simulink model "sys_sim_whx"  (R2023b)
settings: Solver=ode45  StartTime=0.0  StopTime=30  FixedStep=0.001  MaxStep=0.001  MinStep=0.0001  RelTol=1e-3
model workspace (MAT data in the model file):
  Ld = 0.27
  Lu = 0.15
  Tj_MAX = 35
  Tw_MAX = 7
values from neighbouring files (symbols this model uses):
  eta_l = 0.4406    [sys_calc.m]    (also in sys_calc_whx.m = 0.3088)
  g = 9.80665    [sys_calc.m]    (also in sys_calc_whx.m)
  mb = 18.3393    [sys_calc.m]
  ml = 0.924    [sys_calc.m]
  N = NM + mp*diff(x + L*sin(theta),t,2)    [sys_calc_whx.m]
  Rl = 0.18    [sys_calc.m]
  Rw = 0.06    [sys_calc.m]
undefined symbols (not defined in the file or in its folder): X, Y, Z
libraries: sm_lib x76, nesl_utility x38, simulink x9, slpidlib x4
(part 1 of 4)
settings Model: SimulationMode=accelerator  Creator=XH  LastModifiedBy=XHServer
settings DataIOCC: ReturnWorkspaceOutputs=off
settings OptimizationCC: ReuseModelBlockBuffer=off
settings DebuggingCC: ReadBeforeWriteMsg=DisableAll  WriteAfterWriteMsg=DisableAll  WriteAfterReadMsg=DisableAll  MultiTaskDSMMsg=none
settings ModelReferenceCC: UpdateModelReferenceTargets=IfOutOfDate  EnableParallelModelReferenceBuilds=on
settings SFSimCC: SFSimEcho=off  SimTargetLang=C++
settings ExplorerConfigSet: InternalSimMechanicsExplorerSettings="<ExplorerConfiguration><canonicalview>planar_xy</canonicalview><AnimationSetting><BasePlaybackSpeed>1.0</BasePlaybackSpeed><PlaybackSpeedFactor>1.0</PlaybackSpeedFactor></AnimationSetting><TilePanel><TileInfo><Tiles Columns=\"1\" Count=\"1\" Rows=\"1\"><Column Weight=\"1\"/><Row Weight=\"1\"/><Tile Height=\"1\" Width=\"1\" X=\"0\" Y=\"0\"/></Tiles></TileInfo><SceneInfo><SceneViewer><BGColor><R>0.60000002384185791</R><G>0.60000002384185791</G><B>0.60000002384185791</B></BGColor><Camera><DoPerspective>off</DoPerspective><Position><X>8.61621392892213223</X><Y>7.77837481059580949</Y><Z>8.14104102643142014</Z></Position><Center><X>0.437671063196747923</X><Y>-0.400168055129575428</Y><Z>-0.0375018392939591994</Z></Center><Up><X>-0.408248290463863073</X><Y>0.816496580927726145</Y><Z>-0.408248290463863073</Z></Up><ViewLimDist>1</ViewLimDist><YLim>4.22529414972195827</YLim><XLim>7.13870261586088883</XLim></Camera></SceneViewer></SceneInfo></TilePanel><MechEditorPanel><Cameras/><GfxPanelCameraMap/><VideoCreator><PlaybackSpeedRatio>1.0</PlaybackSpeedRatio><FrameRate>30</FrameRate><VideoFormat>Motion JPEG AVI</VideoFormat><FrameSize>auto</FrameSize></VideoCreator></MechEditorPanel></ExplorerConfiguration>"

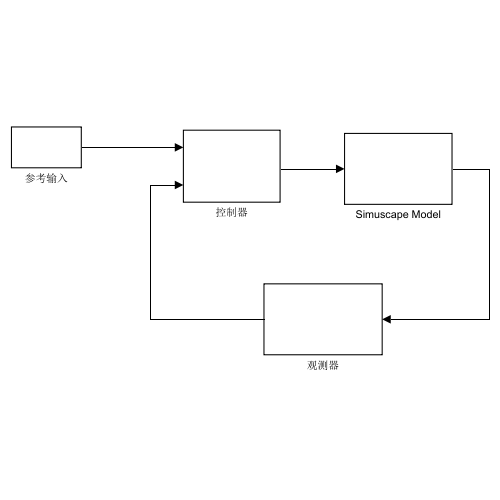
[thumbnail: Simulink's stored preview of the top-level diagram]
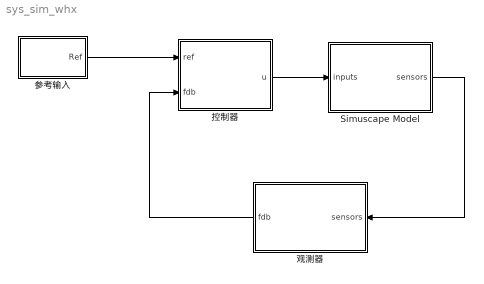
== system sys_sim_whx ==
  Simuscape Model : Subsystem
  参考输入 : Subsystem
  控制器 : Subsystem
  观测器 : Subsystem
  wires:
  Simuscape Model/1(sensors) -> 观测器/1(sensors)
  观测器/1(fdb) -> 控制器/2(fdb)
  参考输入/1(Ref) -> 控制器/1(ref)
  控制器/1(u) -> Simuscape Model/1(inputs)

== system sys_sim_whx/Simuscape Model ==
  inputs : Inport
  Bus Creator : BusCreator  Inputs=28
  Bus Selector1 : BusSelector  OutputSignals=T_lwl,T_lwr,T_Jl1,T_Jl2,T_Jr1,T_Jr2
  Physical System : Subsystem
  sensors : Outport
  wires:
  Bus Selector1/5 -> Physical System/5(T_Jr1)  "<T_Jr1>"
  Bus Selector1/6 -> Physical System/6(T_Jr2)  "<T_Jr2>"
  Bus Selector1/4 -> Physical System/4(T_Jl2)  "<T_Jl2>"
  Bus Selector1/3 -> Physical System/3(T_Jl1)  "<T_Jl1>"
  Bus Selector1/1 -> Physical System/1(T_lwl)  "<T_lwl>"
  Bus Selector1/2 -> Physical System/2(T_lwr)  "<T_lwr>"
  Bus Creator/1 -> sensors/1
  inputs/1 -> Bus Selector1/1
  Physical System/17(Φd) -> Bus Creator/17  "Φd"
  Physical System/16(Φ) -> Bus Creator/16  "Φ"
  Physical System/15(θ_wr) -> Bus Creator/15  "θ_wr"
  Physical System/14(θ_wrd) -> Bus Creator/14  "θ_wrd"
  Physical System/13(θ_wl) -> Bus Creator/13  "θ_wl"
  Physical System/12(θ_wld) -> Bus Creator/12  "θ_wld"
  Physical System/11(θ_Jr2) -> Bus Creator/11  "θ_Jr2"
  Physical System/10(θ_Jr1) -> Bus Creator/10  "θ_Jr1"
  Physical System/9(θ_Jl2) -> Bus Creator/9  "θ_Jl2"
  Physical System/8(θ_Jl1) -> Bus Creator/8  "θ_Jl1"
  Physical System/7(lr) -> Bus Creator/7  "lr"
  Physical System/6(θ_blr) -> Bus Creator/6  "θ_blr"
  Physical System/5(ll) -> Bus Creator/5  "ll"
  Physical System/4(θ_bll) -> Bus Creator/4  "θ_bll"
  Physical System/3(ψ) -> Bus Creator/3  "ψ"
  Physical System/2(θ_bd) -> Bus Creator/2  "θ_bd"
  Physical System/1(θ_b) -> Bus Creator/1  "θ_b"
  Physical System/18(s) -> Bus Creator/18  "s"
  Physical System/19(sd) -> Bus Creator/19  "sd"
  Physical System/20(az) -> Bus Creator/20  "az"
  Physical System/21(Tr1) -> Bus Creator/21  "Tr1"
  Physical System/22(Tr2) -> Bus Creator/22  "Tr2"
  Physical System/23(Tl1) -> Bus Creator/23  "Tl1"
  Physical System/24(Tl2) -> Bus Creator/24  "Tl2"
  Physical System/25(θd_Jr1) -> Bus Creator/25  "θd_Jr1"
  Physical System/26(θd_Jr2) -> Bus Creator/26  "θd_Jr2"
  Physical System/27(θd_Jl1) -> Bus Creator/27  "θd_Jl1"
  Physical System/28(θd_Jl2) -> Bus Creator/28  "θd_Jl2"

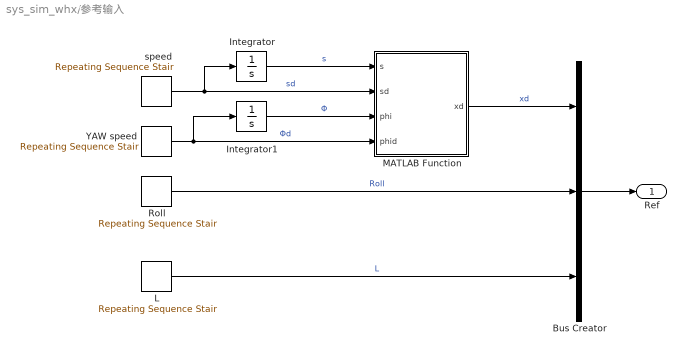
== system sys_sim_whx/参考输入 ==
  Bus Creator : BusCreator  Inputs=3
  Integrator : Integrator
  Integrator1 : Integrator
  L : simulink/Sources/Repeating Sequence Stair  OutValues=[0.2].'  tsamp=2  OutMin=[]  OutMax=[]  OutDataTypeStr=double  OutputDataTypeScalingMode=double  OutDataType=fixdt(0,8)  ConRadixGroup=Best Precision: Vector-wise  OutScaling=2^-12
  MATLAB Function : MATLAB Function  TreatAsAtomicUnit=on
  Roll : simulink/Sources/Repeating Sequence Stair  OutValues=[0].'  tsamp=2  OutMin=[]  OutMax=[]  OutDataTypeStr=double  OutputDataTypeScalingMode=double  OutDataType=fixdt(0,8)  ConRadixGroup=Best Precision: Vector-wise  OutScaling=2^-12
  YAW speed : simulink/Sources/Repeating Sequence Stair  OutValues=[0 ].'  tsamp=2  OutMin=[]  OutMax=[]  OutDataTypeStr=double  OutputDataTypeScalingMode=double  OutDataType=fixdt(0,8)  ConRadixGroup=Best Precision: Vector-wise  OutScaling=2^-12
  speed : simulink/Sources/Repeating Sequence Stair  OutValues=[0 0 -1 0 0].'  tsamp=2  OutMin=[]  OutMax=[]  OutDataTypeStr=double  OutputDataTypeScalingMode=double  OutDataType=fixdt(0,8)  ConRadixGroup=Best Precision: Vector-wise  OutScaling=2^-12
  Ref : Outport
  wires:
  YAW speed/1 -> MATLAB Function/4(phid), Integrator1/1  "Φd"
  speed/1 -> MATLAB Function/2(sd), Integrator/1  "sd"
  Bus Creator/1 -> Ref/1
  MATLAB Function/1(xd) -> Bus Creator/1  "xd"
  Roll/1 -> Bus Creator/2  "Roll"
  L/1 -> Bus Creator/3  "L"
  Integrator1/1 -> MATLAB Function/3(phi)  "Φ"
  Integrator/1 -> MATLAB Function/1(s)  "s"

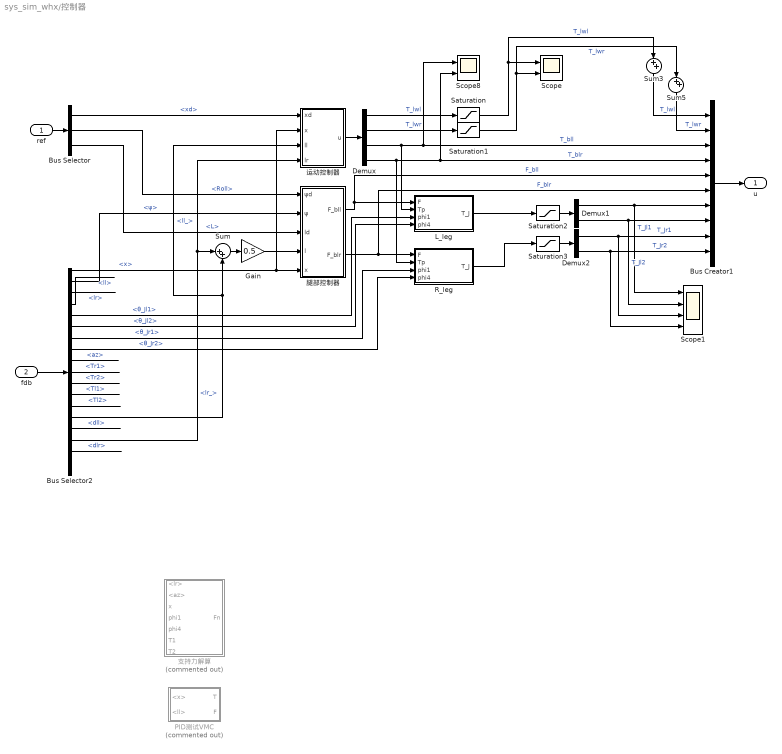
== system sys_sim_whx/控制器 ==
  ref : Inport
  fdb : Inport  Port=2
  Bus Creator1 : BusCreator  Inputs=10
  Bus Selector : BusSelector  OutputSignals=xd,Roll,L
  Bus Selector2 : BusSelector  OutputSignals=x,ψ,ll,lr,θ_Jl1,θ_Jl2,θ_Jr1,θ_Jr2,az,Tr1,Tr2,Tl1,Tl2,ll_,dll,lr_,dlr,θ_wld,θ_wrd
  Demux : Demux
  Demux1 : Demux  Outputs=2
  Demux2 : Demux  Outputs=2
  Gain : Gain  Gain=0.5
  L_leg : MATLAB Function  TreatAsAtomicUnit=on
  PID测试VMC : Subsystem  Commented=on
  R_leg : MATLAB Function  TreatAsAtomicUnit=on
  Saturation : Saturate  UpperLimit=Tw_MAX  LowerLimit=-Tw_MAX  ZeroCross=off
  Saturation1 : Saturate  UpperLimit=Tw_MAX  LowerLimit=-Tw_MAX  ZeroCross=off
  Saturation2 : Saturate  UpperLimit=Tj_MAX  LowerLimit=-Tj_MAX  ZeroCross=off
  Saturation3 : Saturate  UpperLimit=Tj_MAX  LowerLimit=-Tj_MAX  ZeroCross=off
  Scope : Scope  NumInputPorts=2
  Scope1 : Scope  NumInputPorts=4
  Scope8 : Scope  NumInputPorts=2
  Sum : Sum  Inputs=|++
  Sum3 : Sum  Inputs=|++
  Sum5 : Sum  Inputs=|++
  支持力解算 : Subsystem  Commented=on
  腿部控制器 : Subsystem
  运动控制器 : Subsystem
  u : Outport
  wires:
  腿部控制器/2(F_blr) -> R_leg/1(F), Bus Creator1/6  "F_blr"
  Bus Selector2/7 -> R_leg/3(phi1)  "<θ_Jr1>"
  Bus Selector/1 -> 运动控制器/1(xd)  "<xd>"
  Bus Selector2/1 -> 腿部控制器/5(x), 运动控制器/2(x)  "<x>"
  Gain/1 -> 腿部控制器/4(l)
  Demux1/2 -> Bus Creator1/8, Scope1/2  "T_Jl2"
  Sum/1 -> Gain/1
  Demux1/1 -> Scope1/1, Bus Creator1/7  "T_Jl1"
  腿部控制器/1(F_bll) -> L_leg/1(F), Bus Creator1/5  "F_bll"
  ref/1 -> Bus Selector/1
  Bus Selector/2 -> 腿部控制器/1(ψd)  "<Roll>"
  运动控制器/1(u) -> Demux/1
  Bus Selector2/8 -> R_leg/4(phi4)  "<θ_Jr2>"
  fdb/1 -> Bus Selector2/1
  Demux2/1 -> Scope1/3, Bus Creator1/9  "T_Jr1"
  Demux2/2 -> Scope1/4, Bus Creator1/10  "T_Jr2"
  Bus Creator1/1 -> u/1
  Saturation/1 -> Sum3/1, Scope/1  "T_lwl"
  Saturation1/1 -> Scope/2, Sum5/1  "T_lwr"
  Demux/1 -> Saturation/1  "T_lwl"
  Demux/2 -> Saturation1/1  "T_lwr"
  L_leg/1(T_J) -> Saturation2/1
  R_leg/1(T_J) -> Saturation3/1
  Bus Selector2/5 -> L_leg/3(phi1)  "<θ_Jl1>"
  Bus Selector2/6 -> L_leg/4(phi4)  "<θ_Jl2>"
  Demux/4 -> R_leg/2(Tp), Scope8/2, Bus Creator1/4  "T_blr"
  Demux/3 -> L_leg/2(Tp), Scope8/1, Bus Creator1/3  "T_bll"
  Saturation3/1 -> Demux2/1
  Saturation2/1 -> Demux1/1
  Bus Selector/3 -> 腿部控制器/3(ld)  "<L>"
  Bus Selector2/17 -> ?  "<dlr>"
  Bus Selector2/15 -> ?  "<dll>"
  Bus Selector2/2 -> 腿部控制器/2(ψ)  "<ψ>"
  Bus Selector2/9 -> ?  "<az>"
  Bus Selector2/10 -> ?  "<Tr1>"
  Bus Selector2/11 -> ?  "<Tr2>"
  Bus Selector2/12 -> ?  "<Tl1>"
  Bus Selector2/13 -> ?  "<Tl2>"
  Bus Selector2/14 -> 运动控制器/3(ll), Sum/2  "<ll_>"
  Bus Selector2/16 -> Sum/1, 运动控制器/4(lr)  "<lr_>"
  Bus Selector2/3 -> ?  "<ll>"
  Bus Selector2/4 -> ?  "<lr>"
  Sum5/1 -> Bus Creator1/2  "T_lwr"
  Sum3/1 -> Bus Creator1/1  "T_lwl"

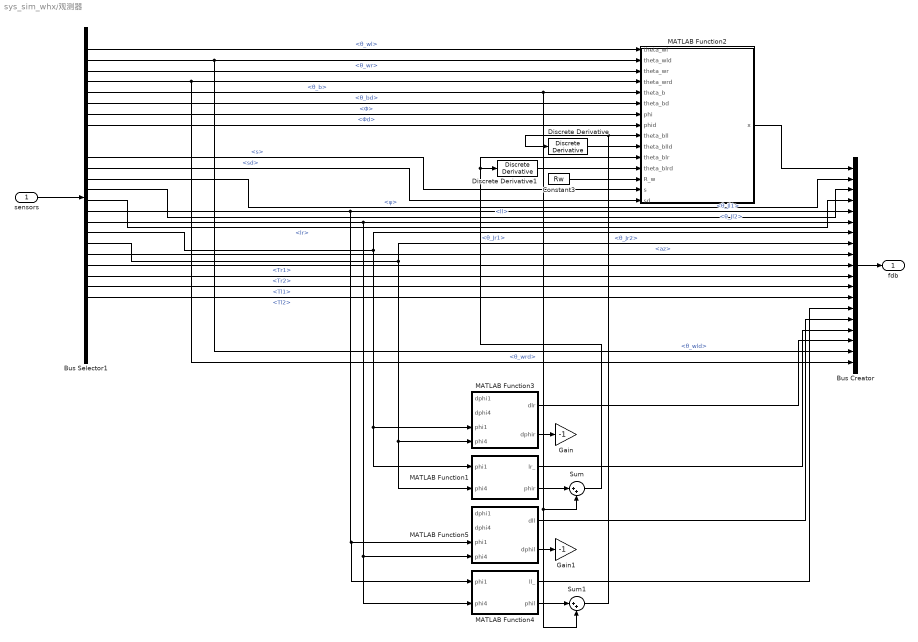
== system sys_sim_whx/观测器 ==
  sensors : Inport
  Bus Creator : BusCreator  Inputs=19
  Bus Selector1 : BusSelector  OutputSignals=θ_wl,θ_wld,θ_wr,θ_wrd,θ_b,θ_bd,Φ,Φd,θ_bll,θ_blr,s,sd,ψ,ll,lr,θ_Jl1,θ_Jl2,θ_Jr1,θ_Jr2,az,Tr1,Tr2,Tl1,Tl2,θd_Jr1,θd_Jr2,θd_Jl1,θd_Jl2
  Constant3 : Constant  Value=Rw
  Discrete Derivative : simulink/Discrete/Discrete Derivative  gainval=1.0  ICPrevScaledInput=0.0  OutMin=[]  OutMax=[]  OutDataType=fixdt(1, 16)  OutScaling=2^-10  DoSatur=off
  Discrete Derivative1 : simulink/Discrete/Discrete Derivative  gainval=1.0  ICPrevScaledInput=0.0  OutMin=[]  OutMax=[]  OutDataType=fixdt(1, 16)  OutScaling=2^-10  DoSatur=off
  Gain : Gain  Gain=-1
  Gain1 : Gain  Gain=-1
  MATLAB Function1 : MATLAB Function  TreatAsAtomicUnit=on
  MATLAB Function2 : MATLAB Function  TreatAsAtomicUnit=on
  MATLAB Function3 : MATLAB Function  TreatAsAtomicUnit=on
  MATLAB Function4 : MATLAB Function  TreatAsAtomicUnit=on
  MATLAB Function5 : MATLAB Function  TreatAsAtomicUnit=on
  Sum : Sum  Inputs=|++
  Sum1 : Sum  Inputs=|++
  fdb : Outport
  wires:
  Constant3/1 -> MATLAB Function2/13(R_w)
  Bus Selector1/1 -> MATLAB Function2/1(theta_wl)  "<θ_wl>"
  Bus Selector1/19 -> MATLAB Function1/2(phi4), MATLAB Function3/4(phi4), Bus Creator/8  "<θ_Jr2>"
  Bus Selector1/17 -> MATLAB Function4/2(phi4), MATLAB Function5/4(phi4), Bus Creator/6  "<θ_Jl2>"
  Bus Selector1/6 -> MATLAB Function2/6(theta_bd)  "<θ_bd>"
  Bus Selector1/4 -> MATLAB Function2/4(theta_wrd), Bus Creator/19  "<θ_wrd>"
  MATLAB Function2/1(x) -> Bus Creator/1
  Bus Selector1/2 -> Bus Creator/18, MATLAB Function2/2(theta_wld)  "<θ_wld>"
  Bus Selector1/3 -> MATLAB Function2/3(theta_wr)  "<θ_wr>"
  Bus Selector1/18 -> MATLAB Function1/1(phi1), MATLAB Function3/3(phi1), Bus Creator/7  "<θ_Jr1>"
  Bus Selector1/13 -> Bus Creator/2  "<ψ>"
  Bus Selector1/14 -> Bus Creator/3  "<ll>"
  Bus Creator/1 -> fdb/1
  Bus Selector1/7 -> MATLAB Function2/7(phi)  "<Φ>"
  Bus Selector1/16 -> MATLAB Function4/1(phi1), MATLAB Function5/3(phi1), Bus Creator/5  "<θ_Jl1>"
  Bus Selector1/5 -> MATLAB Function2/5(theta_b), Sum1/2, Sum/2  "<θ_b>"
  Bus Selector1/8 -> MATLAB Function2/8(phid)  "<Φd>"
  Bus Selector1/15 -> Bus Creator/4  "<lr>"
  sensors/1 -> Bus Selector1/1
  Bus Selector1/11 -> MATLAB Function2/14(s)  "<s>"
  Bus Selector1/12 -> MATLAB Function2/15(sd)  "<sd>"
  Bus Selector1/20 -> Bus Creator/9  "<az>"
  Bus Selector1/21 -> Bus Creator/10  "<Tr1>"
  Bus Selector1/22 -> Bus Creator/11  "<Tr2>"
  Bus Selector1/23 -> Bus Creator/12  "<Tl1>"
  Bus Selector1/24 -> Bus Creator/13  "<Tl2>"
  MATLAB Function4/1(ll_) -> Bus Creator/14
  MATLAB Function5/1(dll) -> Bus Creator/15
  MATLAB Function1/1(lr_) -> Bus Creator/16
  MATLAB Function3/1(dlr) -> Bus Creator/17
  MATLAB Function3/2(dphir) -> Gain/1
  MATLAB Function5/2(dphil) -> Gain1/1
  MATLAB Function1/2(phir) -> Sum/1
  MATLAB Function4/2(phil) -> Sum1/1
  Sum/1 -> Discrete Derivative1/1, MATLAB Function2/11(theta_blr)
  Sum1/1 -> MATLAB Function2/9(theta_bll), Discrete Derivative/1
  Discrete Derivative/1 -> MATLAB Function2/10(theta_blld)
  Discrete Derivative1/1 -> MATLAB Function2/12(theta_blrd)

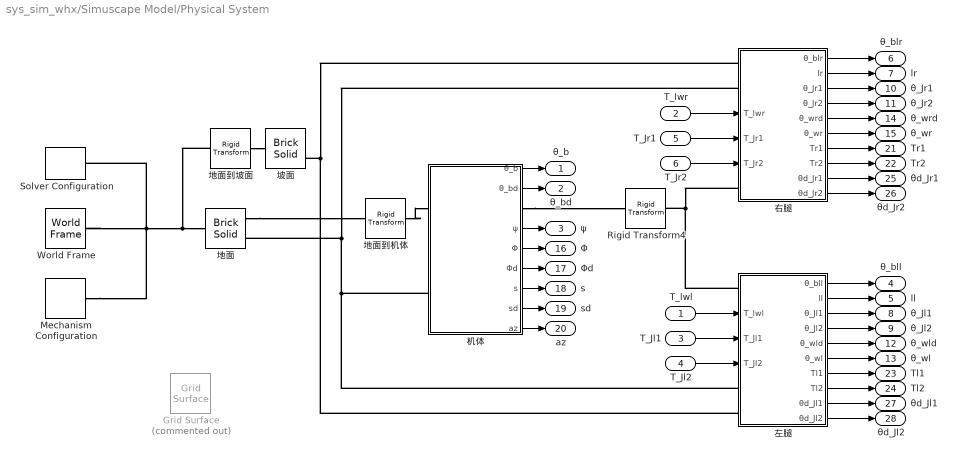
== system sys_sim_whx/Simuscape Model/Physical System ==
  T_lwl : Inport
  T_lwr : Inport  Port=2
  T_Jl1 : Inport  Port=3
  T_Jl2 : Inport  Port=4
  T_Jr1 : Inport  Port=5
  T_Jr2 : Inport  Port=6
  Grid Surface : sm_lib/Curves and Surfaces/Grid Surface  Commented=on  XGridVector=[0 1 2 3]  XGridVectorUnits=m  YGridVector=[0 1 2 3]  YGridVectorUnits=m  ZHeights=[0 0 .5 .5; 0 0 .5 .5; 0 0 0 0; 0 0 0 0]  ZHeightsUnits=m  GraphicType=FromGeometry  GraphicVisPropType=SimpleVisualProperties  GraphicDiffuseColor=[0.5 0.5 0.5]  GraphicOpacity=1.0  GraphicSpecularColor=[0.5 0.5 0.5 1.0]  GraphicAmbientColor=[0.15 0.15 0.15 1.0]  GraphicEmissiveColor=[0.0 0.0 0.0 1.0]  GraphicShininess=75
  Mechanism Configuration : sm_lib/Utilities/Mechanism Configuration  UniformGravity=Constant  GravityVector=[0 -9.80665 0]  GravityVectorUnits=m/s^2  LinearizationDelta=0.001  JointModeTransitionNonlinearIterations=2
  Rigid Transform4 : sm_lib/Frames and Transforms/Rigid Transform  TranslationMethod=StandardAxis  TranslationStandardOffset=0.02  TranslationStandardOffsetUnits=m  TranslationStandardAxis=-Y  TranslationCartesianOffset=[0 0 0]  TranslationCartesianOffsetUnits=m  TranslationROffset=0  TranslationROffsetUnits=m  TranslationZOffset=0  TranslationZOffsetUnits=m  TranslationThetaOffset=0  TranslationThetaOffsetUnits=deg  RotationMethod=None  RotationAngleUnits=deg  RotationStandardAxis=+Z  RotationAngle=0.0  RotationArbitraryAxis=[0 0 1]  FollAlignAxisA=+X  BaseAlignAxisA=+Y  FollAlignAxisB=+Y  BaseAlignAxisB=+Z  RotationSequenceAxes=FollowerAxes  RotationSequence=XYX  RotationSequenceAngles=[0 0 0]  RotationSequenceAnglesUnits=deg  RotationMatrix=[1 0 0; 0 1 0; 0 0 1]  Quaternion=[1 0 0 0]
  Solver Configuration : nesl_utility/Solver Configuration  PhysicalDomain=network_engine_domain  SubClassName=solver  LeftPortType=input  RightPortType=generic  Tones=[]  Harmonics=[]  SimulateNoise=off  Profile=off  UseLocalSampling=off  EnableSwitchedLinearOptims=on  FrequencyDomain=off  UseCCode=off  RelTol=0.001  AbsTol=1e-06  MinStep=1e-09  ToWorkspace=off  RevertToSquareIcSolve=off  NumHomotopyIterations=100  PhasorMode=off  PhasorModeNumHarmonics=1  ConsistencySolver=NEWTON_XTOL_AFTER_FTOL  IndexReductionMethod=DerivativeReplacement  DoDC=off  ResidualTolerance=1e-09  ConsistencyTolSource=GLOBAL  ConsistencyAbsTol=0.001  ConsistencyRelTol=0.001  ConsistencyTolFactor=0.001  UseLocalSolver=off  LocalSolverChoice=NE_BACKWARD_EULER_ADVANCER  ResolveIndetEquations=on  FunctionEvalNumThread=1  LocalSolverSampleTime=0.001  DoFixedCost=off  MaxNonlinIter=3  MaxModeIter=2  ComputeImpulses=off  ImpulseIterations=2  LinearAlgebra=Sparse  LinearAlgebraNumThread=0  EquationFormulation=NE_TIME_EF  DelaysMemoryBudget=1024  AutomaticFiltering=on  FilteringTimeConstant=0.001  PartitionStorageMethod=AS_NEEDED  PartitionMemoryBudget=1024  PartitionMethod=FAST  MultibodyUseLocalSolver=off  MultibodyLocalSolverChoice=ODE1  MultibodyLocalSolverSampleTime=0.001
  World Frame : sm_lib/Frames and Transforms/World Frame
  右腿 : Subsystem
      settings: PortSchema="{\"entries\":[{\"content\":{\"sides\":[{\"content\":{\"connectorIds\":[\"LConn1\",\"LConn2\",\"In1\",\"In2\",\"In3\",\"LConn3\"]},\"type\":\"ConnectorPlacement.EquallySpacedRectSide\",\"uuid\":\"e2ccd12d-a564-41f8-9643-0a0e2b5d7e59\"},{\"content\":{\"connectorIds\":[\"Out1\",\"Out2\",\"Out3\",\"Out4\",\"Out5\",\"Out6\",\"Out7\",\"Out8\",\"Out9\",\"Out10\"],\"side\":\"RIGHT\"},\"type\":\"ConnectorPlacement.EquallySpacedRectSide\",\"uuid\":\"2e2dbfb9-e5d7-4b1e-ae3e-ddd297310d21\"},{\"content\":{\"side\":\"TOP\"},\"type\":\"ConnectorPlacement.EquallySpacedRectSide\",\"uuid\":\"1bb563b8-e4fe-4d0e-86bd-84293b91cae2\"}]},\"type\":\"ConnectorPlacement.EquallySpacedConnector\",\"uuid\":\"35c068bd-e6d2-480e-9c80-85749dea9d4d\"}],\"packageUris\":[\"http://schema.mathworks.com/mf0/Connector/R2020b\"],\"version\":\"1.0\"}"
  地面 : sm_lib/Body Elements/Brick Solid  GraphicAmbientColor=[0.3 0.3 0.3 1.0]  BasedOnType=Density  BrickDimensions=[200 0.05 20]  BrickDimensionsUnits=m  CenterOfMass=[0 0 0]  CenterOfMassUnits=m  GraphicDiffuseColor=[0.5 0.5 0.5]  Density=1000  DensityUnits=kg/m^3  DoExposeReferenceFrame=on  GraphicEmissiveColor=[0.0 0.0 0.0 1.0]  ExportEntireGeometry=on  SerializedFrames=<Frames><Frame><Id>Frame1</Id><Value><Name>F1</Name><Origin><Source>ReferenceFrame</Source><FeatureName></FeatureName></Origin><PrimaryAxis><DefinedDirection>+Z</DefinedDirection><Source>ReferenceFrame</Source><SourceDirection>+Z</SourceDirection><FeatureName></FeatureName></PrimaryAxis><SecondaryAxis><DefinedDirection>+X</DefinedDirection><Source>ReferenceFrame</Source><SourceDirection>+X</SourceDirection><FeatureName></FeatureName></SecondaryAxis></Value></Frame></Frames>  MarkerShape=Sphere  MarkerSize=10  GraphicType=FromGeometry  InertiaType=CalculateFromGeometry  Mass=1  MassUnits=kg  MomentsOfInertia=[1 1 1]  MomentsOfInertiaUnits=kg*m^2  GraphicOpacity=1  ProductsOfInertia=[0 0 0]  ProductsOfInertiaUnits=kg*m^2  GraphicShininess=20  GraphicSpecularColor=[0.9 0.9 0.9 1.0]  GraphicVisPropType=AdvancedVisualProperties
  地面到坡面 : sm_lib/Frames and Transforms/Rigid Transform  TranslationMethod=StandardAxis  TranslationStandardOffset=2  TranslationStandardOffsetUnits=m  TranslationStandardAxis=+X  TranslationCartesianOffset=[0 0 0]  TranslationCartesianOffsetUnits=m  TranslationROffset=0  TranslationROffsetUnits=m  TranslationZOffset=0  TranslationZOffsetUnits=m  TranslationThetaOffset=0  TranslationThetaOffsetUnits=deg  RotationMethod=StandardAxis  RotationAngleUnits=deg  RotationStandardAxis=+Z  RotationAngle=17  RotationArbitraryAxis=[0 0 1]  FollAlignAxisA=+X  BaseAlignAxisA=+Y  FollAlignAxisB=+Y  BaseAlignAxisB=+Z  RotationSequenceAxes=FollowerAxes  RotationSequence=XYX  RotationSequenceAngles=[0 0 0]  RotationSequenceAnglesUnits=deg  RotationMatrix=[1 0 0; 0 1 0; 0 0 1]  Quaternion=[1 0 0 0]
  地面到机体 : sm_lib/Frames and Transforms/Rigid Transform  TranslationMethod=StandardAxis  TranslationStandardOffset=0.24  TranslationStandardOffsetUnits=m  TranslationStandardAxis=+Y  TranslationCartesianOffset=[0 0 0]  TranslationCartesianOffsetUnits=m  TranslationROffset=0  TranslationROffsetUnits=m  TranslationZOffset=0  TranslationZOffsetUnits=m  TranslationThetaOffset=0  TranslationThetaOffsetUnits=deg  RotationMethod=None  RotationAngleUnits=deg  RotationStandardAxis=+Z  RotationAngle=5  RotationArbitraryAxis=[0 0 1]  FollAlignAxisA=+X  BaseAlignAxisA=+Y  FollAlignAxisB=+Y  BaseAlignAxisB=+Z  RotationSequenceAxes=FollowerAxes  RotationSequence=XYX  RotationSequenceAngles=[0 0 0]  RotationSequenceAnglesUnits=deg  RotationMatrix=[1 0 0; 0 1 0; 0 0 1]  Quaternion=[1 0 0 0]
  坡面 : sm_lib/Body Elements/Brick Solid  GraphicAmbientColor=[0.3 0.3 0.3 1.0]  BasedOnType=Density  BrickDimensions=[2.406 0.05 2]  BrickDimensionsUnits=m  CenterOfMass=[0 0 0]  CenterOfMassUnits=m  GraphicDiffuseColor=[0.5 0.5 0.5]  Density=1000  DensityUnits=kg/m^3  DoExposeReferenceFrame=on  GraphicEmissiveColor=[0.0 0.0 0.0 1.0]  ExportEntireGeometry=on  SerializedFrames=<Frames><Frame><Id>Frame1</Id><Value><Name>F1</Name><Origin><Source>ReferenceFrame</Source><FeatureName></FeatureName></Origin><PrimaryAxis><DefinedDirection>+Z</DefinedDirection><Source>ReferenceFrame</Source><SourceDirection>+Z</SourceDirection><FeatureName></FeatureName></PrimaryAxis><SecondaryAxis><DefinedDirection>+X</DefinedDirection><Source>ReferenceFrame</Source><SourceDirection>+X</SourceDirection><FeatureName></FeatureName></SecondaryAxis></Value></Frame></Frames>  MarkerShape=Sphere  MarkerSize=10  GraphicType=FromGeometry  InertiaType=CalculateFromGeometry  Mass=1  MassUnits=kg  MomentsOfInertia=[1 1 1]  MomentsOfInertiaUnits=kg*m^2  GraphicOpacity=1  ProductsOfInertia=[0 0 0]  ProductsOfInertiaUnits=kg*m^2  GraphicShininess=20  GraphicSpecularColor=[0.9 0.9 0.9 1.0]  GraphicVisPropType=AdvancedVisualProperties
  左腿 : Subsystem
      settings: PortSchema="{\"entries\":[{\"content\":{\"sides\":[{\"content\":{\"connectorIds\":[\"LConn1\",\"In1\",\"In2\",\"In3\",\"LConn2\",\"LConn3\"]},\"type\":\"ConnectorPlacement.EquallySpacedRectSide\",\"uuid\":\"e2ccd12d-a564-41f8-9643-0a0e2b5d7e59\"},{\"content\":{\"connectorIds\":[\"Out1\",\"Out2\",\"Out3\",\"Out4\",\"Out5\",\"Out6\",\"Out7\",\"Out8\",\"Out9\",\"Out10\"],\"side\":\"RIGHT\"},\"type\":\"ConnectorPlacement.EquallySpacedRectSide\",\"uuid\":\"2e2dbfb9-e5d7-4b1e-ae3e-ddd297310d21\"},{\"content\":{\"side\":\"TOP\"},\"type\":\"ConnectorPlacement.EquallySpacedRectSide\",\"uuid\":\"1bb563b8-e4fe-4d0e-86bd-84293b91cae2\"}]},\"type\":\"ConnectorPlacement.EquallySpacedConnector\",\"uuid\":\"35c068bd-e6d2-480e-9c80-85749dea9d4d\"}],\"packageUris\":[\"http://schema.mathworks.com/mf0/Connector/R2020b\"],\"version\":\"1.0\"}"
  机体 : Subsystem
      settings: PortSchema="{\"entries\":[{\"content\":{\"sides\":[{\"content\":{\"connectorIds\":[\"LConn1\",\"LConn2\"]},\"type\":\"ConnectorPlacement.EquallySpacedRectSide\",\"uuid\":\"d45d031a-c7d7-48c1-917a-e164a86c5711\"},{\"content\":{\"connectorIds\":[\"Out1\",\"Out2\",\"RConn1\",\"Out3\",\"Out4\",\"Out5\",\"Out6\",\"Out7\",\"Out8\"],\"side\":\"RIGHT\"},\"type\":\"ConnectorPlacement.EquallySpacedRectSide\",\"uuid\":\"8e2629e6-a512-4ae9-87f8-c479e3d4ffb0\"},{\"content\":{\"side\":\"TOP\"},\"type\":\"ConnectorPlacement.EquallySpacedRectSide\",\"uuid\":\"87919977-2508-495d-8de8-0bc18e999a2c\"}]},\"type\":\"ConnectorPlacement.EquallySpacedConnector\",\"uuid\":\"7dfad816-ad42-4a41-b9b6-f645954b83c1\"}],\"packageUris\":[\"http://schema.mathworks.com/mf0/Connector/R2020b\"],\"version\":\"1.0\"}"
  θ_b : Outport
  θ_bd : Outport  Port=2
  ψ : Outport  Port=3
  θ_bll : Outport  Port=4
  ll : Outport  Port=5
  θ_blr : Outport  Port=6
  lr : Outport  Port=7
  θ_Jl1 : Outport  Port=8
  θ_Jl2 : Outport  Port=9
  θ_Jr1 : Outport  Port=10
  θ_Jr2 : Outport  Port=11
  θ_wld : Outport  Port=12
  θ_wl : Outport  Port=13
  θ_wrd : Outport  Port=14
  θ_wr : Outport  Port=15
  Φ : Outport  Port=16
  Φd : Outport  Port=17
  s : Outport  Port=18
  sd : Outport  Port=19
  az : Outport  Port=20
  Tr1 : Outport  Port=21
  Tr2 : Outport  Port=22
  Tl1 : Outport  Port=23
  Tl2 : Outport  Port=24
  θd_Jr1 : Outport  Port=25
  θd_Jr2 : Outport  Port=26
  θd_Jl1 : Outport  Port=27
  θd_Jl2 : Outport  Port=28
  wires:
  T_lwl/1 -> 左腿/1(T_lwl)
  T_Jl1/1 -> 左腿/2(T_Jl1)
  T_Jl2/1 -> 左腿/3(T_Jl2)
  左腿/1(θ_bll) -> θ_bll/1
  左腿/2(ll) -> ll/1
  左腿/3(θ_Jl1) -> θ_Jl1/1
  左腿/4(θ_Jl2) -> θ_Jl2/1
  左腿/5(θ_wld) -> θ_wld/1
  左腿/6(θ_wl) -> θ_wl/1
  T_lwr/1 -> 右腿/1(T_lwr)
  T_Jr1/1 -> 右腿/2(T_Jr1)
  T_Jr2/1 -> 右腿/3(T_Jr2)
  右腿/1(θ_blr) -> θ_blr/1
  右腿/2(lr) -> lr/1
  右腿/3(θ_Jr1) -> θ_Jr1/1
  右腿/4(θ_Jr2) -> θ_Jr2/1
  右腿/5(θ_wrd) -> θ_wrd/1
  右腿/6(θ_wr) -> θ_wr/1
  机体/1(θ_b) -> θ_b/1
  机体/2(θ_bd) -> θ_bd/1
  机体/3(ψ) -> ψ/1
  机体/4(Φ) -> Φ/1
  机体/5(Φd) -> Φd/1
  机体/6(s) -> s/1
  机体/7(sd) -> sd/1
  机体/8(az) -> az/1
  右腿/7(Tr1) -> Tr1/1
  右腿/8(Tr2) -> Tr2/1
  左腿/7(Tl1) -> Tl1/1
  左腿/8(Tl2) -> Tl2/1
  右腿/10(θd_Jr2) -> θd_Jr2/1
  右腿/9(θd_Jr1) -> θd_Jr1/1
  左腿/9(θd_Jl1) -> θd_Jl1/1
  左腿/10(θd_Jl2) -> θd_Jl2/1
  connections:
  地面/LConn2 -- 右腿/LConn2 -- 机体/LConn2 -- 左腿/LConn2
  左腿/LConn1 -- 右腿/LConn3 -- Rigid Transform4/RConn1
  机体/RConn1 -- Rigid Transform4/LConn1
  地面到机体/RConn1 -- 机体/LConn1
  地面/LConn1 -- 地面到机体/LConn1
  地面到坡面/RConn1 -- 坡面/RConn1
  World Frame/RConn1 -- 地面到坡面/LConn1 -- 地面/RConn1 -- Mechanism Configuration/RConn1 -- Solver Configuration/RConn1
  右腿/LConn1 -- 左腿/LConn3 -- 坡面/LConn2

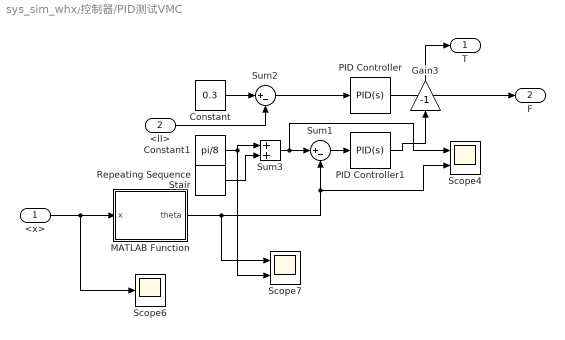
== system sys_sim_whx/控制器/PID测试VMC ==
  <x> : Inport
  <ll> : Inport  Port=2
  Constant : Constant  Value=0.3
  Constant1 : Constant  Value=pi/8
  Gain3 : Gain  Gain=-1
  MATLAB Function : MATLAB Function  TreatAsAtomicUnit=on
  PID Controller : slpidlib/PID Controller  Controller=PID  Form=Parallel  TimeDomain=Continuous-time  UseExternalTs=off  SampleTime=-1  IntegratorMethod=Forward Euler  FilterMethod=Forward Euler  ControllerParametersSource=internal  P=8000  I=1000  UseKiTs=off  D=1000  N=100  UseFilter=on  TunerSelectOption=Transfer Function Based (PID Tuner App)  InitialConditionSource=internal  InitialConditionForIntegrator=0  InitialConditionForFilter=0  DifferentiatorICPrevScaledInput=0  ExternalReset=none  TrackingMode=off  Kt=1  LimitOutput=off  SatLimitsSource=internal  UpperSaturationLimit=inf  LowerSaturationLimit=-inf  LinearizeAsGain=on  AntiWindupMode=none  Kb=1  LimitIntegrator=off  UpperIntegratorSaturationLimit=inf  LowerIntegratorSaturationLimit=-inf  POutMin=[]  POutMax=[]  IOutMin=[]  IOutMax=[]  DOutMin=[]  DOutMax=[]  NOutMin=[]  NOutMax=[]  SumOutMin=[]  SumOutMax=[]  SaturationOutMin=[]  SaturationOutMax=[]  PParamMin=[]  PParamMax=[]  IParamMin=[]  IParamMax=[]  DParamMin=[]  DParamMax=[]  NParamMin=[]  NParamMax=[]  KbParamMin=[]  KbParamMax=[]  KtParamMin=[]  KtParamMax=[]  KbOutMin=[]  KbOutMax=[]  KtOutMin=[]  KtOutMax=[]  IntegratorOutMin=[]  IntegratorOutMax=[]  FilterOutMin=[]  FilterOutMax=[]  SumI1OutMin=[]  SumI1OutMax=[]  SumI2OutMin=[]  SumI2OutMax=[]  SumI3OutMin=[]  SumI3OutMax=[]  SumI4OutMin=[]  SumI4OutMax=[]  SumDOutMin=[]  SumDOutMax=[]  DifferentiatorOutMin=[]  DifferentiatorOutMax=[]  FilterDiffOutCoefMin=[]  FilterDiffOutCoefMax=[]  ReciprocalOutMin=[]  ReciprocalOutMax=[]  SumDenOutMin=[]  SumDenOutMax=[]  SumNumOutMin=[]  SumNumOutMax=[]  DivideOutMin=[]  DivideOutMax=[]  UdiffTsProdOutMin=[]  UdiffTsProdOutMax=[]  NTsProdOutMin=[]  NTsProdOutMax=[]  UintegralTsProdOutMin=[]  UintegralTsProdOutMax=[]  UngainTsProdOutMin=[]  UngainTsProdOutMax=[]  ClampingZeroOutDataTypeStr=Inherit: Inherit via back propagation  ClampingZeroOutMin=[]  ClampingZeroOutMax=[]  FilterDenConstantOutDataTypeStr=Inherit: Inherit via back propagation  FilterDenConstantOutMin=[]  FilterDenConstantOutMax=[]  PCopyOutDataTypeStr=Inherit: Inherit via back propagation  PCopyOutMin=[]  PCopyOutMax=[]  NCopyOutDataTypeStr=Inherit: Inherit via back propagation  NCopyOutMin=[]  NCopyOutMax=[]  IntegratorContinuousStateAttributes=''  IntegratorStateMustResolveToSignalObject=off  IntegratorRTWStateStorageClass=Auto  FilterContinuousStateAttributes=''  FilterStateMustResolveToSignalObject=off  FilterRTWStateStorageClass=Auto  ParallelPVariant=InternalParameters  IdealPVariant=Disabled  IVariant=InternalParameters  DVariant=InternalParameters  IntegratorVariant=Continuous  SatVariant=Disabled  AWVariant=Passthrough  PCopyVariant=Disabled  TRVariant=Disabled  FdbkBlocksVariant=Forward  IdealPFdbkVariant=Disabled  SatFdbkVariant=Disabled  DerivativeFilterVariant=ContFilter  NVariant=InternalParameters  NCopyVariant=Disabled  FilterICVariant=InternalICsFilter  IntegratorICVariant=InternalICs  ExternalResetVariant=Disabled  TRSumVariant=Passthrough  SumFdbkVariant=Disabled  SumVariant=Sum_PID  TsampFilterVariant=InternalTs  TsampNgainVariant=Passthrough  TsampIntegralVariant=Disabled_SignalSpec  ExternalSaturationOutDataTypeStr=Inherit: Same as second input
  PID Controller1 : slpidlib/PID Controller  Controller=PID  Form=Parallel  TimeDomain=Continuous-time  UseExternalTs=off  SampleTime=-1  IntegratorMethod=Forward Euler  FilterMethod=Forward Euler  ControllerParametersSource=internal  P=1000  I=0  UseKiTs=off  D=0  N=100  UseFilter=on  TunerSelectOption=Transfer Function Based (PID Tuner App)  InitialConditionSource=internal  InitialConditionForIntegrator=0  InitialConditionForFilter=0  DifferentiatorICPrevScaledInput=0  ExternalReset=none  TrackingMode=off  Kt=1  LimitOutput=off  SatLimitsSource=internal  UpperSaturationLimit=inf  LowerSaturationLimit=-inf  LinearizeAsGain=on  AntiWindupMode=none  Kb=1  LimitIntegrator=off  UpperIntegratorSaturationLimit=inf  LowerIntegratorSaturationLimit=-inf  POutMin=[]  POutMax=[]  IOutMin=[]  IOutMax=[]  DOutMin=[]  DOutMax=[]  NOutMin=[]  NOutMax=[]  SumOutMin=[]  SumOutMax=[]  SaturationOutMin=[]  SaturationOutMax=[]  PParamMin=[]  PParamMax=[]  IParamMin=[]  IParamMax=[]  DParamMin=[]  DParamMax=[]  NParamMin=[]  NParamMax=[]  KbParamMin=[]  KbParamMax=[]  KtParamMin=[]  KtParamMax=[]  KbOutMin=[]  KbOutMax=[]  KtOutMin=[]  KtOutMax=[]  IntegratorOutMin=[]  IntegratorOutMax=[]  FilterOutMin=[]  FilterOutMax=[]  SumI1OutMin=[]  SumI1OutMax=[]  SumI2OutMin=[]  SumI2OutMax=[]  SumI3OutMin=[]  SumI3OutMax=[]  SumI4OutMin=[]  SumI4OutMax=[]  SumDOutMin=[]  SumDOutMax=[]  DifferentiatorOutMin=[]  DifferentiatorOutMax=[]  FilterDiffOutCoefMin=[]  FilterDiffOutCoefMax=[]  ReciprocalOutMin=[]  ReciprocalOutMax=[]  SumDenOutMin=[]  SumDenOutMax=[]  SumNumOutMin=[]  SumNumOutMax=[]  DivideOutMin=[]  DivideOutMax=[]  UdiffTsProdOutMin=[]  UdiffTsProdOutMax=[]  NTsProdOutMin=[]  NTsProdOutMax=[]  UintegralTsProdOutMin=[]  UintegralTsProdOutMax=[]  UngainTsProdOutMin=[]  UngainTsProdOutMax=[]  ClampingZeroOutDataTypeStr=Inherit: Inherit via back propagation  ClampingZeroOutMin=[]  ClampingZeroOutMax=[]  FilterDenConstantOutDataTypeStr=Inherit: Inherit via back propagation  FilterDenConstantOutMin=[]  FilterDenConstantOutMax=[]  PCopyOutDataTypeStr=Inherit: Inherit via back propagation  PCopyOutMin=[]  PCopyOutMax=[]  NCopyOutDataTypeStr=Inherit: Inherit via back propagation  NCopyOutMin=[]  NCopyOutMax=[]  IntegratorContinuousStateAttributes=''  IntegratorStateMustResolveToSignalObject=off  IntegratorRTWStateStorageClass=Auto  FilterContinuousStateAttributes=''  FilterStateMustResolveToSignalObject=off  FilterRTWStateStorageClass=Auto  ParallelPVariant=InternalParameters  IdealPVariant=Disabled  IVariant=InternalParameters  DVariant=InternalParameters  IntegratorVariant=Continuous  SatVariant=Disabled  AWVariant=Passthrough  PCopyVariant=Disabled  TRVariant=Disabled  FdbkBlocksVariant=Forward  IdealPFdbkVariant=Disabled  SatFdbkVariant=Disabled  DerivativeFilterVariant=ContFilter  NVariant=InternalParameters  NCopyVariant=Disabled  FilterICVariant=InternalICsFilter  IntegratorICVariant=InternalICs  ExternalResetVariant=Disabled  TRSumVariant=Passthrough  SumFdbkVariant=Disabled  SumVariant=Sum_PID  TsampFilterVariant=InternalTs  TsampNgainVariant=Passthrough  TsampIntegralVariant=Disabled_SignalSpec  ExternalSaturationOutDataTypeStr=Inherit: Same as second input
  Repeating Sequence Stair : simulink/Sources/Repeating Sequence Stair  OutValues=[0 -pi/8 -pi/4].'  tsamp=1  OutMin=[]  OutMax=[]  OutDataTypeStr=double  OutputDataTypeScalingMode=double  OutDataType=fixdt(0,8)  ConRadixGroup=Best Precision: Vector-wise  OutScaling=2^-12
  Scope4 : Scope  NumInputPorts=2
  Scope6 : Scope
  Scope7 : Scope  NumInputPorts=2
  Sum1 : Sum  Inputs=|+-
  Sum2 : Sum  Inputs=|+-
  Sum3 : Sum  Inputs=|++
  T : Outport
  F : Outport  Port=2
  wires:
  Constant1/1 -> Scope7/2, Sum3/1
  <ll>/1 -> Sum2/2
  PID Controller1/1 -> Gain3/1
  <x>/1 -> MATLAB Function/1(x), Scope6/1
  Sum2/1 -> PID Controller/1
  Sum3/1 -> Scope4/1, Sum1/1
  MATLAB Function/1(theta) -> Scope4/2, Sum1/2, Scope7/1
  Repeating Sequence Stair/1 -> Sum3/2
  Constant/1 -> Sum2/1
  Sum1/1 -> PID Controller1/1
  PID Controller/1 -> F/1
  Gain3/1 -> T/1

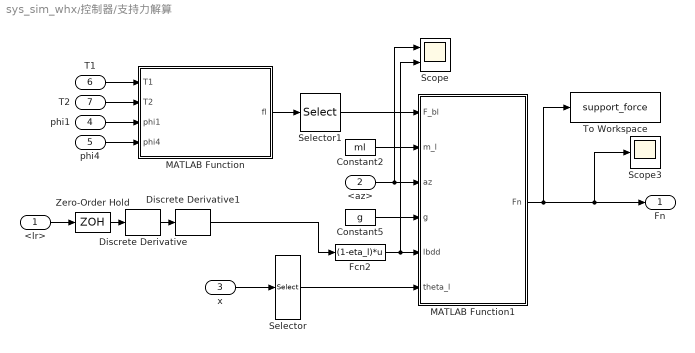
== system sys_sim_whx/控制器/支持力解算 ==
  <lr> : Inport
  <az> : Inport  Port=2
  x : Inport  Port=3
  phi1 : Inport  Port=4
  phi4 : Inport  Port=5
  T1 : Inport  Port=6
  T2 : Inport  Port=7
  Constant2 : Constant  Value=ml
  Constant5 : Constant  Value=g
  Discrete Derivative : simulink/Discrete/Discrete Derivative  gainval=1.0  ICPrevScaledInput=0.0  OutMin=[]  OutMax=[]  OutDataType=fixdt(1, 16)  OutScaling=2^-10  DoSatur=off
  Discrete Derivative1 : simulink/Discrete/Discrete Derivative  gainval=1.0  ICPrevScaledInput=0.0  OutMin=[]  OutMax=[]  OutDataType=fixdt(1, 16)  OutScaling=2^-10  DoSatur=off
  Fcn2 : Fcn  Expr=(1-eta_l)*u
  MATLAB Function : MATLAB Function  TreatAsAtomicUnit=on
  MATLAB Function1 : MATLAB Function  TreatAsAtomicUnit=on
  Scope : Scope  NumInputPorts=2
  Scope3 : Scope
  Selector : Selector  InputPortWidth=10  IndexOptions=Index vector (dialog)  Indices=7  OutputSizes=1
  Selector1 : Selector  InputPortWidth=2  IndexOptions=Index vector (dialog)  Indices=1  OutputSizes=1
  To Workspace : ToWorkspace  VariableName=support_force  SaveFormat=Timeseries  SampleTime=-1
  Zero-Order Hold : ZeroOrderHold  SampleTime=0.001
  Fn : Outport
  wires:
  Constant5/1 -> MATLAB Function1/4(g)
  Constant2/1 -> MATLAB Function1/2(m_l)
  <az>/1 -> Scope/1, MATLAB Function1/3(az)
  Fcn2/1 -> Scope/2, MATLAB Function1/5(lbdd)
  Selector/1 -> MATLAB Function1/6(theta_l)
  x/1 -> Selector/1
  <lr>/1 -> Zero-Order Hold/1
  Zero-Order Hold/1 -> Discrete Derivative/1
  Discrete Derivative/1 -> Discrete Derivative1/1
  Discrete Derivative1/1 -> Fcn2/1
  MATLAB Function1/1(Fn) -> Fn/1, Scope3/1, To Workspace/1
  phi1/1 -> MATLAB Function/3(phi1)
  phi4/1 -> MATLAB Function/4(phi4)
  T1/1 -> MATLAB Function/1(T1)
  T2/1 -> MATLAB Function/2(T2)
  MATLAB Function/1(fl) -> Selector1/1
  Selector1/1 -> MATLAB Function1/1(F_bl)

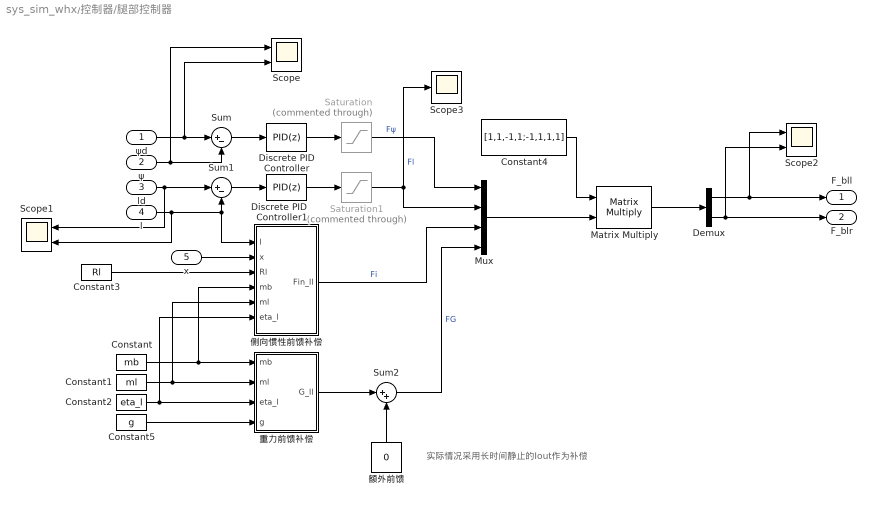
== system sys_sim_whx/控制器/腿部控制器 ==
  note: 实际情况采用长时间静止的Iout作为补偿
  ψd : Inport
  ψ : Inport  Port=2
  ld : Inport  Port=3
  l : Inport  Port=4
  x : Inport  Port=5
  Constant : Constant  Value=mb
  Constant1 : Constant  Value=ml
  Constant2 : Constant  Value=eta_l
  Constant3 : Constant  Value=Rl
  Constant4 : Constant  Value=[1,1,-1,1;-1,1,1,1]
  Constant5 : Constant  Value=g
  Demux : Demux  Outputs=2
  Discrete PID Controller : slpidlib/PID Controller  Controller=PID  Form=Parallel  TimeDomain=Discrete-time  UseExternalTs=off  SampleTime=0.001  IntegratorMethod=Forward Euler  FilterMethod=Forward Euler  ControllerParametersSource=internal  P=300  I=0  UseKiTs=off  D=0  N=100  UseFilter=on  TunerSelectOption=Transfer Function Based (PID Tuner App)  InitialConditionSource=internal  InitialConditionForIntegrator=0  InitialConditionForFilter=0  DifferentiatorICPrevScaledInput=0  ExternalReset=none  TrackingMode=off  Kt=1  LimitOutput=off  SatLimitsSource=internal  UpperSaturationLimit=inf  LowerSaturationLimit=-inf  LinearizeAsGain=off  AntiWindupMode=none  Kb=1  LimitIntegrator=off  UpperIntegratorSaturationLimit=inf  LowerIntegratorSaturationLimit=-inf  POutMin=[]  POutMax=[]  IOutMin=[]  IOutMax=[]  DOutMin=[]  DOutMax=[]  NOutMin=[]  NOutMax=[]  SumOutMin=[]  SumOutMax=[]  SaturationOutMin=[]  SaturationOutMax=[]  PParamMin=[]  PParamMax=[]  IParamMin=[]  IParamMax=[]  DParamMin=[]  DParamMax=[]  NParamMin=[]  NParamMax=[]  KbParamMin=[]  KbParamMax=[]  KtParamMin=[]  KtParamMax=[]  KbOutMin=[]  KbOutMax=[]  KtOutMin=[]  KtOutMax=[]  IntegratorOutMin=[]  IntegratorOutMax=[]  FilterOutMin=[]  FilterOutMax=[]  SumI1OutMin=[]  SumI1OutMax=[]  SumI2OutMin=[]  SumI2OutMax=[]  SumI3OutMin=[]  SumI3OutMax=[]  SumI4OutMin=[]  SumI4OutMax=[]  SumDOutMin=[]  SumDOutMax=[]  DifferentiatorOutMin=[]  DifferentiatorOutMax=[]  FilterDiffOutCoefMin=[]  FilterDiffOutCoefMax=[]  ReciprocalOutMin=[]  ReciprocalOutMax=[]  SumDenOutMin=[]  SumDenOutMax=[]  SumNumOutMin=[]  SumNumOutMax=[]  DivideOutMin=[]  DivideOutMax=[]  UdiffTsProdOutMin=[]  UdiffTsProdOutMax=[]  NTsProdOutMin=[]  NTsProdOutMax=[]  UintegralTsProdOutMin=[]  UintegralTsProdOutMax=[]  UngainTsProdOutMin=[]  UngainTsProdOutMax=[]  ClampingZeroOutDataTypeStr=Inherit: Inherit via back propagation  ClampingZeroOutMin=[]  ClampingZeroOutMax=[]  FilterDenConstantOutDataTypeStr=Inherit: Inherit via back propagation  FilterDenConstantOutMin=[]  FilterDenConstantOutMax=[]  PCopyOutDataTypeStr=Inherit: Inherit via back propagation  PCopyOutMin=[]  PCopyOutMax=[]  NCopyOutDataTypeStr=Inherit: Inherit via back propagation  NCopyOutMin=[]  NCopyOutMax=[]  IntegratorContinuousStateAttributes=''  IntegratorStateMustResolveToSignalObject=off  IntegratorRTWStateStorageClass=Auto  FilterContinuousStateAttributes=''  FilterStateMustResolveToSignalObject=off  FilterRTWStateStorageClass=Auto  ParallelPVariant=InternalParameters  IdealPVariant=Disabled  IVariant=InternalParameters  DVariant=InternalParameters  IntegratorVariant=Discrete  SatVariant=Disabled  AWVariant=Passthrough  PCopyVariant=Disabled  TRVariant=Disabled  FdbkBlocksVariant=Forward  IdealPFdbkVariant=Disabled  SatFdbkVariant=Disabled  DerivativeFilterVariant=ForwardEulerFilter  NVariant=InternalParameters  NCopyVariant=Disabled  FilterICVariant=InternalICsFilter  IntegratorICVariant=InternalICs  ExternalResetVariant=Disabled  TRSumVariant=Passthrough  SumFdbkVariant=Disabled  SumVariant=Sum_PID  TsampFilterVariant=InternalTs  TsampNgainVariant=Passthrough  TsampIntegralVariant=Disabled_SignalSpec  ExternalSaturationOutDataTypeStr=Inherit: Same as second input
      settings: LibrarySourceBlock=simulink/Discrete/Discrete PID Controller
  Discrete PID Controller1 : slpidlib/PID Controller  Controller=PID  Form=Parallel  TimeDomain=Discrete-time  UseExternalTs=off  SampleTime=0.001  IntegratorMethod=Forward Euler  FilterMethod=Forward Euler  ControllerParametersSource=internal  P=3000  I=50  UseKiTs=off  D=60  N=100  UseFilter=on  TunerSelectOption=Transfer Function Based (PID Tuner App)  InitialConditionSource=internal  InitialConditionForIntegrator=0  InitialConditionForFilter=0  DifferentiatorICPrevScaledInput=0  ExternalReset=none  TrackingMode=off  Kt=1  LimitOutput=off  SatLimitsSource=internal  UpperSaturationLimit=inf  LowerSaturationLimit=-inf  LinearizeAsGain=off  AntiWindupMode=none  Kb=1  LimitIntegrator=off  UpperIntegratorSaturationLimit=inf  LowerIntegratorSaturationLimit=-inf  POutMin=[]  POutMax=[]  IOutMin=[]  IOutMax=[]  DOutMin=[]  DOutMax=[]  NOutMin=[]  NOutMax=[]  SumOutMin=[]  SumOutMax=[]  SaturationOutMin=[]  SaturationOutMax=[]  PParamMin=[]  PParamMax=[]  IParamMin=[]  IParamMax=[]  DParamMin=[]  DParamMax=[]  NParamMin=[]  NParamMax=[]  KbParamMin=[]  KbParamMax=[]  KtParamMin=[]  KtParamMax=[]  KbOutMin=[]  KbOutMax=[]  KtOutMin=[]  KtOutMax=[]  IntegratorOutMin=[]  IntegratorOutMax=[]  FilterOutMin=[]  FilterOutMax=[]  SumI1OutMin=[]  SumI1OutMax=[]  SumI2OutMin=[]  SumI2OutMax=[]  SumI3OutMin=[]  SumI3OutMax=[]  SumI4OutMin=[]  SumI4OutMax=[]  SumDOutMin=[]  SumDOutMax=[]  DifferentiatorOutMin=[]  DifferentiatorOutMax=[]  FilterDiffOutCoefMin=[]  FilterDiffOutCoefMax=[]  ReciprocalOutMin=[]  ReciprocalOutMax=[]  SumDenOutMin=[]  SumDenOutMax=[]  SumNumOutMin=[]  SumNumOutMax=[]  DivideOutMin=[]  DivideOutMax=[]  UdiffTsProdOutMin=[]  UdiffTsProdOutMax=[]  NTsProdOutMin=[]  NTsProdOutMax=[]  UintegralTsProdOutMin=[]  UintegralTsProdOutMax=[]  UngainTsProdOutMin=[]  UngainTsProdOutMax=[]  ClampingZeroOutDataTypeStr=Inherit: Inherit via back propagation  ClampingZeroOutMin=[]  ClampingZeroOutMax=[]  FilterDenConstantOutDataTypeStr=Inherit: Inherit via back propagation  FilterDenConstantOutMin=[]  FilterDenConstantOutMax=[]  PCopyOutDataTypeStr=Inherit: Inherit via back propagation  PCopyOutMin=[]  PCopyOutMax=[]  NCopyOutDataTypeStr=Inherit: Inherit via back propagation  NCopyOutMin=[]  NCopyOutMax=[]  IntegratorContinuousStateAttributes=''  IntegratorStateMustResolveToSignalObject=off  IntegratorRTWStateStorageClass=Auto  FilterContinuousStateAttributes=''  FilterStateMustResolveToSignalObject=off  FilterRTWStateStorageClass=Auto  ParallelPVariant=InternalParameters  IdealPVariant=Disabled  IVariant=InternalParameters  DVariant=InternalParameters  IntegratorVariant=Discrete  SatVariant=Disabled  AWVariant=Passthrough  PCopyVariant=Disabled  TRVariant=Disabled  FdbkBlocksVariant=Forward  IdealPFdbkVariant=Disabled  SatFdbkVariant=Disabled  DerivativeFilterVariant=ForwardEulerFilter  NVariant=InternalParameters  NCopyVariant=Disabled  FilterICVariant=InternalICsFilter  IntegratorICVariant=InternalICs  ExternalResetVariant=Disabled  TRSumVariant=Passthrough  SumFdbkVariant=Disabled  SumVariant=Sum_PID  TsampFilterVariant=InternalTs  TsampNgainVariant=Passthrough  TsampIntegralVariant=Disabled_SignalSpec  ExternalSaturationOutDataTypeStr=Inherit: Same as second input
      settings: LibrarySourceBlock=simulink/Discrete/Discrete PID Controller
  Matrix Multiply : Product  Multiplication=Matrix(*)
  Mux : Mux
  Saturation : Saturate  Commented=through
  Saturation1 : Saturate  Commented=through
  Scope : Scope  NumInputPorts=2
  Scope1 : Scope  NumInputPorts=2
  Scope2 : Scope  NumInputPorts=2
  Scope3 : Scope
  Sum : Sum  Inputs=|+-
  Sum1 : Sum  Inputs=|+-
  Sum2 : Sum  Inputs=|++
  侧向惯性前馈补偿 : MATLAB Function  TreatAsAtomicUnit=on
  重力前馈补偿 : MATLAB Function  TreatAsAtomicUnit=on
  额外前馈 : Constant  Value=0
  F_bll : Outport
  F_blr : Outport  Port=2
  wires:
  Saturation/1 -> Mux/1  "Fψ"
  Discrete PID Controller/1 -> Saturation/1
  ld/1 -> Scope1/1, Sum1/1
  ψ/1 -> Scope/1, Sum/2
  Constant/1 -> 侧向惯性前馈补偿/4(mb), 重力前馈补偿/1(mb)
  l/1 -> 侧向惯性前馈补偿/1(l), Sum1/2, Scope1/2
  ψd/1 -> Scope/2, Sum/1
  Saturation1/1 -> Mux/2, Scope3/1  "Fl"
  Sum/1 -> Discrete PID Controller/1
  Mux/1 -> Matrix Multiply/2
  Constant2/1 -> 侧向惯性前馈补偿/6(eta_l), 重力前馈补偿/3(eta_l)
  Demux/1 -> Scope2/1, F_bll/1
  Demux/2 -> Scope2/2, F_blr/1
  Constant4/1 -> Matrix Multiply/1
  Constant3/1 -> 侧向惯性前馈补偿/3(Rl)
  Constant1/1 -> 侧向惯性前馈补偿/5(ml), 重力前馈补偿/2(ml)
  x/1 -> 侧向惯性前馈补偿/2(x)
  Constant5/1 -> 重力前馈补偿/4(g)
  重力前馈补偿/1(G_ll) -> Sum2/1
  Sum2/1 -> Mux/4  "FG"
  额外前馈/1 -> Sum2/2
  Matrix Multiply/1 -> Demux/1
  侧向惯性前馈补偿/1(Fin_ll) -> Mux/3  "Fi"
  Discrete PID Controller1/1 -> Saturation1/1
  Sum1/1 -> Discrete PID Controller1/1

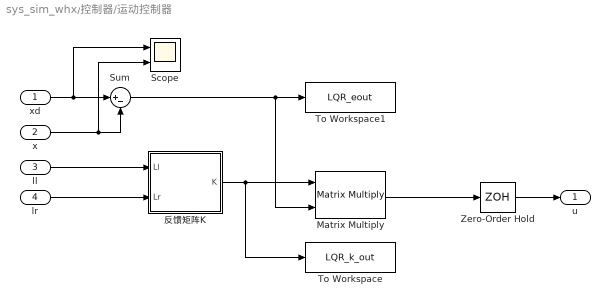
== system sys_sim_whx/控制器/运动控制器 ==
  xd : Inport
  x : Inport  Port=2
  ll : Inport  Port=3
  lr : Inport  Port=4
  Matrix Multiply : Product  Multiplication=Matrix(*)
  Scope : Scope  NumInputPorts=2
  Sum : Sum  Inputs=|+-
  To Workspace : ToWorkspace  VariableName=LQR_k_out  SaveFormat=Timeseries  SampleTime=-1
  To Workspace1 : ToWorkspace  VariableName=LQR_eout  SaveFormat=Timeseries  SampleTime=-1
  Zero-Order Hold : ZeroOrderHold  SampleTime=0.001
  反馈矩阵K : MATLAB Function  TreatAsAtomicUnit=on
  u : Outport
  wires:
  x/1 -> Scope/2, Sum/2
  lr/1 -> 反馈矩阵K/2(Lr)
  ll/1 -> 反馈矩阵K/1(Ll)
  反馈矩阵K/1(K) -> To Workspace/1, Matrix Multiply/1
  xd/1 -> Scope/1, Sum/1
  Sum/1 -> Matrix Multiply/2, To Workspace1/1
  Zero-Order Hold/1 -> u/1
  Matrix Multiply/1 -> Zero-Order Hold/1
